simulink model "sim_dist"  (R2020a)
settings: Solver=FixedStepAuto  StartTime=0.0  StopTime=2  FixedStep=0.000001  RelTol=1e-3
undefined symbols (not defined in the file): Clpfdist_z, Gnominal_z
libraries: cstblocks x4
settings Model: Creator=yuimu  LastModifiedBy=yuimu
settings SolverCC: AlgebraicLoopSolver=LineSearch
settings SFSimCC: CustomCodeUndefinedFunction=UseInterfaceOnly

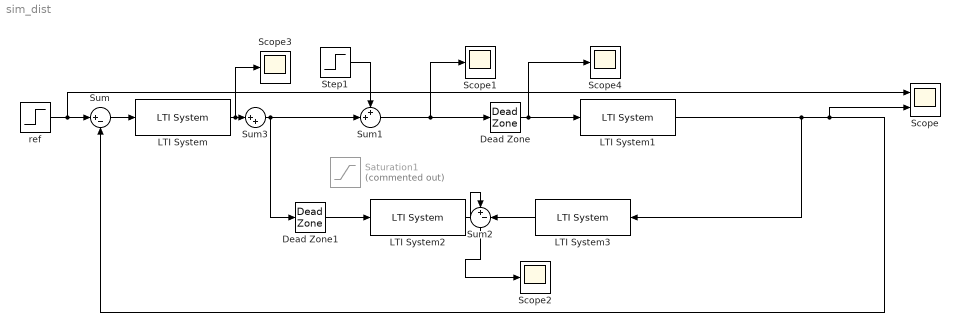
== system sim_dist ==
  Dead Zone : DeadZone  LowerValue=-0.9  UpperValue=0.9  SaturateOnIntegerOverflow=on
  Dead Zone1 : DeadZone  LowerValue=-0.9  UpperValue=0.9  SaturateOnIntegerOverflow=on
  LTI System : cstblocks/LTI System  sys=Cpd_z  IC=[]
  LTI System1 : cstblocks/LTI System  sys=Gnominal_z  IC=[]
  LTI System2 : cstblocks/LTI System  sys=Clpfdist_z  IC=[]
  LTI System3 : cstblocks/LTI System  sys=Clpfdist_z/Gnominal_z  IC=[]
  Saturation1 : Saturate  Commented=on  UpperLimit=5  LowerLimit=-5
  Scope : Scope  NumInputPorts=2
  Scope{1..4} (4 alike) : Scope
  Step1 : Step  SampleTime=0
  Sum : Sum  Inputs=|+-
  Sum1 : Sum  Inputs=++|
  Sum2 : Sum  Inputs=|+-
  Sum3 : Sum  Inputs=|++
  ref : Step  Time=0  After=0  SampleTime=0
  wires:
  Sum/1 -> LTI System/1
  LTI System2/1 -> Sum2/1
  LTI System3/1 -> Sum2/2
  LTI System/1 -> Scope3/1, Sum3/1
  LTI System1/1 -> Scope/2, Sum/2, LTI System3/1
  ref/1 -> Scope/1, Sum/1
  Step1/1 -> Sum1/1
  Sum2/1 -> Scope2/1
  Dead Zone/1 -> Scope4/1, LTI System1/1
  Sum1/1 -> Dead Zone/1, Scope1/1
  Sum3/1 -> Dead Zone1/1, Sum1/2
  Dead Zone1/1 -> LTI System2/1
